simulink model "sf_gfexport"  (R2017b)
settings: Solver=ode45  StartTime=0.0  StopTime=inf  RelTol=1e-3  EnableMultiTasking=on
settings Model: FPTRunName=Active  ExtModeAutoUpdateStatusClock=off  Creator=The MathWorks, Inc.  LastModifiedBy=The MathWorks, Inc.
settings DataIOCC: LimitDataPoints=on  SaveFormat=Array
settings OptimizationCC: BooleanDataType=off  ExpressionDepthLimit=2147483647  InitFltsAndDblsToZero=on  EfficientMapNaN2IntZero=off  LifeSpan=inf
settings DebuggingCC: SignalRangeChecking=warning  SaveWithParameterizedLinksMsg=none  UnderspecifiedInitializationDetection=Classic  MergeDetectMultiDrivingBlocksExec=none  SignalResolutionControl=TryResolveAllWithWarning  MultiTaskDSMMsg=warning  MultiTaskCondExecSysMsg=none  FcnCallInpInsideContextMsg=warning  StateNameClashWarn=warning  StrictBusMsg=None  SFUnexpectedBacktrackingDiag=warning  SFNoUnconditionalDefaultTransitionDiag=warning  SFExecutionAtInitializationDiag=none
settings HardwareCC: ProdBitPerPointer=32  ProdBitPerSizeT=32  ProdBitPerPtrDiffT=32  ProdLargestAtomicFloat=None  ProdIntDivRoundTo=Undefined  ProdEndianess=Unspecified  ProdWordSize=32  ProdHWDeviceType=32-bit Generic  TargetUnknown=on
settings ModelReferenceCC: PropagateSignalLabelsOutOfModel=off
settings SFSimCC: SimParseCustomCode=off
settings CodeAppCC: StateflowObjectComments=on
settings GRTTargetCC: TargetFcnLib=ansi_tfl_tmw.mat  TargetLangStandard=C89/C90 (ANSI)  GeneratePreprocessorConditionals=Disable all  CombineOutputUpdateFcns=off  GRTInterface=on
settings ConfigComp: CovMetricSettings=dcmtr  CovHtmlReporting=on  CovSaveCumulativeToWorkspaceVar=on  CovSaveSingleToWorkspaceVar=on  CovExternalEMLEnable=off  CovSFcnEnable=off

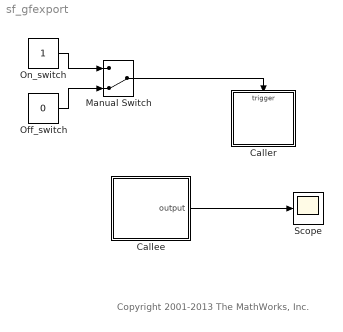
== system sf_gfexport ==
  note: Copyright 2001-2013 The MathWorks, Inc.
  Callee : Stateflow chart  TreatAsAtomicUnit=on
  Caller : Stateflow chart  TreatAsAtomicUnit=on
  Manual Switch : ManualSwitch  CurrentSetting=0
  Off_switch : Constant  Value=0
  On_switch : Constant
  Scope : Scope
  wires:
  On_switch/1 -> Manual Switch/1
  Off_switch/1 -> Manual Switch/2
  Manual Switch/1 -> Caller/Trigger
  Callee/1(output) -> Scope/1

== stateflow chart sf_gfexport/Caller ==
  (default) -> (junction 5)
  (junction 5) -> (junction 4) [order 1] : [is_A_active()]
      | {send_event_to_A();}
  (junction 5) -> (junction 4) [order 2] : {send_event_to_B();}
  events: E input EITHER_EDGE_EVENT

== stateflow chart sf_gfexport/Callee ==
  state B
    entry: output = 1;
  state A
    entry: output = 0;
  state send_event_to_A() [function]
    (default) -> (junction 13) : {send(SWITCH,A);}
  state activity = is_A_active() [function]
    (default) -> (junction 12) : {activity = in(A);}
  state send_event_to_B() [function]
    (default) -> (junction 14) : {send(SWITCH,B);}
  (default) -> A
  B -> A : SWITCH
  A -> B : SWITCH
  data: activity function_output double; output output double
  events: SWITCH local EITHER_EDGE_EVENT
